simulink model "main"  (R2024a)
settings: Solver=VariableStepAuto  StartTime=0.0  StopTime=1  MaxStep=1e-4  RelTol=1e-3
InitFcn:
  | parametros
values from neighbouring files (symbols this model uses):
  alpha_cu = 3.9 *10^-3    (= 0.0039)    [parametros.m]
  b_l = 0.1    [parametros.m]
  b_m = 1.5 * 10^-5    (= 1.5e-05)    [parametros.m]
  C_ts = 0.818    [parametros.m]
  J_l = (m*l_cm^2 + J_cm) + (m_l * l_l^2)    (= 0.0833)    [parametros.m]
  J_m = 1.4 * 10^-5    (= 1.4e-05)    [parametros.m]
  k_l = m * g * l_cm + m_l * g * l_l    (= 2.4516625)    [parametros.m]
  L_d = 6.6 * 10^-3    (= 0.0066)    [parametros.m]
  L_ls = 0.8 * 10^-3    (= 0.0008)    [parametros.m]
  L_q = 5.8 * 10^-3    (= 0.0058)    [parametros.m]
  lambda_m = 0.016    [parametros.m]
  P_p = 3    [parametros.m]
  r = 120    [parametros.m]
  R_s_40 = 1.02    [parametros.m]
  R_ts_amb = 146.7    [parametros.m]
  Temp_s_ref = 40    [parametros.m]
(part 2 of 3)

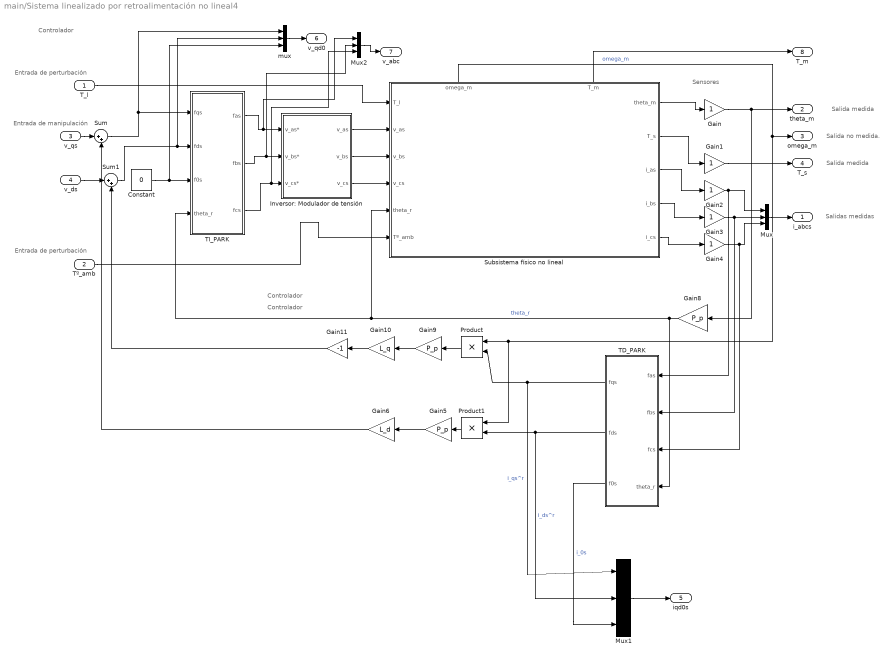
== system main/Sistema linealizado por retroalimentación no lineal4 ==
  note: Entrada de perturbación
  note: Entrada de manipulación
  note: Entrada de perturbación
  note: Controlador
  note: Salida medida
  note: Controlador
  note: Sensores
  note: Salida medida
  note: Salidas medidas
  note: Salida no medida.
  note: Controlador
  T_l : Inport
  Tº_amb : Inport  Port=2
  v_qs : Inport  Port=3
  v_ds : Inport  Port=4
  Constant : Constant  Value=0
  Gain{,1..4} (5 alike) : Gain
  Gain10 : Gain  Gain=L_q
  Gain11 : Gain  Gain=-1
  Gain5 : Gain  Gain=P_p
  Gain6 : Gain  Gain=L_d
  Gain8 : Gain  Gain=P_p
  Gain9 : Gain  Gain=P_p
  Inversor: Modulador de tensión : Subsystem
  Mux : Mux  Inputs=3
  Mux1 : Mux  Inputs=3
  Mux2 : Mux  Inputs=3
  Product : Product
  Product1 : Product
  "Subsistema físico no lineal " : Subsystem
      settings: PortSchema="{\"entries\":[{\"content\":{\"sides\":[{\"content\":{\"connectorIds\":[\"In1\",\"In2\",\"In3\",\"In4\",\"In5\",\"In6\"]},\"type\":\"ConnectorPlacement.EquallySpacedRectSide\",\"uuid\":\"df16c937-5b0d-437b-9581-4e7e4443d731\"},{\"content\":{\"connectorIds\":[\"Out1\",\"Out2\",\"Out3\",\"Out4\",\"Out5\"],\"side\":\"RIGHT\"},\"type\":\"ConnectorPlacement.EquallySpacedRectSide\",\"uuid\":\"58799b56-1bb2-4861-ad63-3fa3f8181ad5\"},{\"content\":{\"connectorIds\":[\"Out6\",\"Out7\"],\"side\":\"TOP\"},\"type\":\"ConnectorPlacement.EquallySpacedRectSide\",\"uuid\":\"9d658df7-49d2-4fa1-a84c-b158d9dac98e\"}]},\"type\":\"ConnectorPlacement.EquallySpacedConnector\",\"uuid\":\"4e139d46-6a94-417e-9cad-9c9676c83a39\"}],\"packageUris\":[\"http://schema.mathworks.com/mf0/Connector/R2020b\"],\"version\":\"1.0\"}"
  Sum : Sum  Inputs=|++
  Sum1 : Sum  Inputs=|++
  TD_PARK : MATLAB Function  TreatAsAtomicUnit=on
  TI_PARK : MATLAB Function  TreatAsAtomicUnit=on
  mux : Mux  Inputs=3
  i_abcs : Outport
  theta_m : Outport  Port=2
  omega_m : Outport  Port=3
  T_s : Outport  Port=4
  iqd0s : Outport  Port=5
  v_qd0 : Outport  Port=6
  v_abc : Outport  Port=7
  T_m : Outport  Port=8
  wires:
  T_l/1 -> "Subsistema físico no lineal "/1(T_l)
  "Subsistema físico no lineal "/2(T_s) -> Gain1/1
  "Subsistema físico no lineal "/1(theta_m) -> Gain/1
  Tº_amb/1 -> "Subsistema físico no lineal "/6(Tº_amb)
  "Subsistema físico no lineal "/4(i_bs) -> Gain3/1
  "Subsistema físico no lineal "/5(i_cs) -> Gain4/1
  "Subsistema físico no lineal "/3(i_as) -> Gain2/1
  Gain2/1 -> TD_PARK/1(fas), Mux/1
  Gain3/1 -> TD_PARK/2(fbs), Mux/2
  Gain4/1 -> TD_PARK/3(fcs), Mux/3
  Mux/1 -> i_abcs/1
  Gain/1 -> Gain8/1, theta_m/1
  "Subsistema físico no lineal "/6(omega_m) -> omega_m/1, Product1/1, Product/1  "omega_m"
  Gain1/1 -> T_s/1
  Gain8/1 -> "Subsistema físico no lineal "/5(theta_r), TI_PARK/4(theta_r), TD_PARK/4(theta_r)  "theta_r"
  TD_PARK/1(fqs) -> Mux1/1, Product/2  "i_qs^r"
  Product/1 -> Gain9/1
  Gain9/1 -> Gain10/1
  Gain10/1 -> Gain11/1
  Constant/1 -> TI_PARK/3(f0s), mux/3
  Inversor: Modulador de tensión/1(v_as) -> "Subsistema físico no lineal "/2(v_as)
  Inversor: Modulador de tensión/2(v_bs) -> "Subsistema físico no lineal "/3(v_bs)
  Inversor: Modulador de tensión/3(v_cs) -> "Subsistema físico no lineal "/4(v_cs)
  TI_PARK/1(fas) -> Mux2/1, Inversor: Modulador de tensión/1(v_as*)
  TI_PARK/2(fbs) -> Mux2/2, Inversor: Modulador de tensión/2(v_bs*)
  TI_PARK/3(fcs) -> Mux2/3, Inversor: Modulador de tensión/3(v_cs*)
  TD_PARK/2(fds) -> Mux1/2, Product1/2  "i_ds^r"
  TD_PARK/3(f0s) -> Mux1/3  "i_0s"
  Product1/1 -> Gain5/1
  Gain5/1 -> Gain6/1
  Mux1/1 -> iqd0s/1
  mux/1 -> v_qd0/1
  Mux2/1 -> v_abc/1
  "Subsistema físico no lineal "/7(T_m) -> T_m/1
  Gain11/1 -> Sum1/2
  v_qs/1 -> Sum/1
  Sum/1 -> TI_PARK/1(fqs), mux/1
  Gain6/1 -> Sum/2
  v_ds/1 -> Sum1/1
  Sum1/1 -> mux/2, TI_PARK/2(fds)

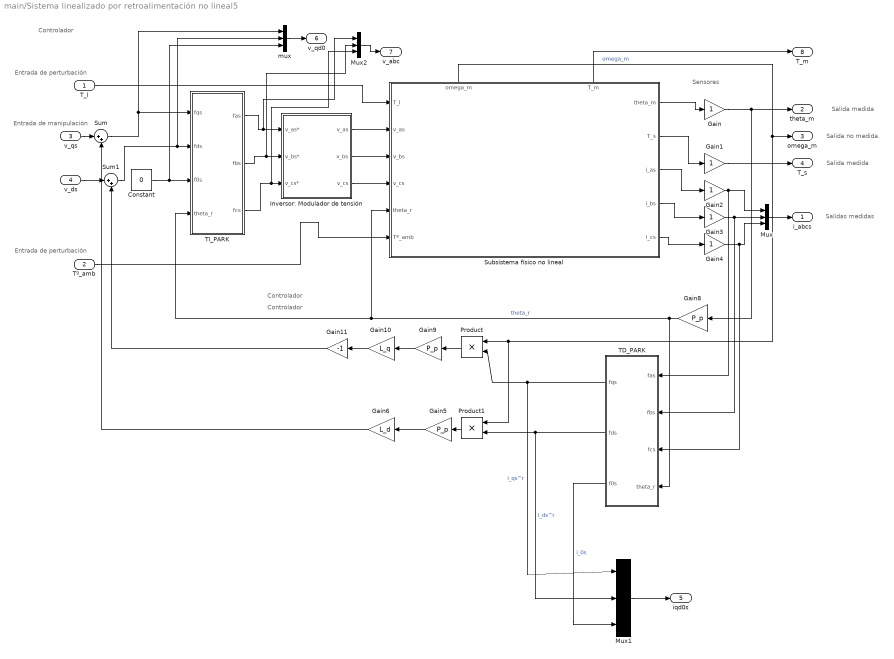
== system main/Sistema linealizado por retroalimentación no lineal5 ==
  note: Entrada de perturbación
  note: Entrada de manipulación
  note: Entrada de perturbación
  note: Controlador
  note: Salida medida
  note: Controlador
  note: Sensores
  note: Salida medida
  note: Salidas medidas
  note: Salida no medida.
  note: Controlador
  T_l : Inport
  Tº_amb : Inport  Port=2
  v_qs : Inport  Port=3
  v_ds : Inport  Port=4
  Constant : Constant  Value=0
  Gain{,1..4} (5 alike) : Gain
  Gain10 : Gain  Gain=L_q
  Gain11 : Gain  Gain=-1
  Gain5 : Gain  Gain=P_p
  Gain6 : Gain  Gain=L_d
  Gain8 : Gain  Gain=P_p
  Gain9 : Gain  Gain=P_p
  Inversor: Modulador de tensión : Subsystem
  Mux : Mux  Inputs=3
  Mux1 : Mux  Inputs=3
  Mux2 : Mux  Inputs=3
  Product : Product
  Product1 : Product
  "Subsistema físico no lineal " : Subsystem
      settings: PortSchema="{\"entries\":[{\"content\":{\"sides\":[{\"content\":{\"connectorIds\":[\"In1\",\"In2\",\"In3\",\"In4\",\"In5\",\"In6\"]},\"type\":\"ConnectorPlacement.EquallySpacedRectSide\",\"uuid\":\"df16c937-5b0d-437b-9581-4e7e4443d731\"},{\"content\":{\"connectorIds\":[\"Out1\",\"Out2\",\"Out3\",\"Out4\",\"Out5\"],\"side\":\"RIGHT\"},\"type\":\"ConnectorPlacement.EquallySpacedRectSide\",\"uuid\":\"58799b56-1bb2-4861-ad63-3fa3f8181ad5\"},{\"content\":{\"connectorIds\":[\"Out6\",\"Out7\"],\"side\":\"TOP\"},\"type\":\"ConnectorPlacement.EquallySpacedRectSide\",\"uuid\":\"9d658df7-49d2-4fa1-a84c-b158d9dac98e\"}]},\"type\":\"ConnectorPlacement.EquallySpacedConnector\",\"uuid\":\"4e139d46-6a94-417e-9cad-9c9676c83a39\"}],\"packageUris\":[\"http://schema.mathworks.com/mf0/Connector/R2020b\"],\"version\":\"1.0\"}"
  Sum : Sum  Inputs=|++
  Sum1 : Sum  Inputs=|++
  TD_PARK : MATLAB Function  TreatAsAtomicUnit=on
  TI_PARK : MATLAB Function  TreatAsAtomicUnit=on
  mux : Mux  Inputs=3
  i_abcs : Outport
  theta_m : Outport  Port=2
  omega_m : Outport  Port=3
  T_s : Outport  Port=4
  iqd0s : Outport  Port=5
  v_qd0 : Outport  Port=6
  v_abc : Outport  Port=7
  T_m : Outport  Port=8
  wires:
  T_l/1 -> "Subsistema físico no lineal "/1(T_l)
  "Subsistema físico no lineal "/2(T_s) -> Gain1/1
  "Subsistema físico no lineal "/1(theta_m) -> Gain/1
  Tº_amb/1 -> "Subsistema físico no lineal "/6(Tº_amb)
  "Subsistema físico no lineal "/4(i_bs) -> Gain3/1
  "Subsistema físico no lineal "/5(i_cs) -> Gain4/1
  "Subsistema físico no lineal "/3(i_as) -> Gain2/1
  Gain2/1 -> TD_PARK/1(fas), Mux/1
  Gain3/1 -> TD_PARK/2(fbs), Mux/2
  Gain4/1 -> TD_PARK/3(fcs), Mux/3
  Mux/1 -> i_abcs/1
  Gain/1 -> Gain8/1, theta_m/1
  "Subsistema físico no lineal "/6(omega_m) -> omega_m/1, Product1/1, Product/1  "omega_m"
  Gain1/1 -> T_s/1
  Gain8/1 -> "Subsistema físico no lineal "/5(theta_r), TI_PARK/4(theta_r), TD_PARK/4(theta_r)  "theta_r"
  TD_PARK/1(fqs) -> Mux1/1, Product/2  "i_qs^r"
  Product/1 -> Gain9/1
  Gain9/1 -> Gain10/1
  Gain10/1 -> Gain11/1
  Constant/1 -> TI_PARK/3(f0s), mux/3
  Inversor: Modulador de tensión/1(v_as) -> "Subsistema físico no lineal "/2(v_as)
  Inversor: Modulador de tensión/2(v_bs) -> "Subsistema físico no lineal "/3(v_bs)
  Inversor: Modulador de tensión/3(v_cs) -> "Subsistema físico no lineal "/4(v_cs)
  TI_PARK/1(fas) -> Mux2/1, Inversor: Modulador de tensión/1(v_as*)
  TI_PARK/2(fbs) -> Mux2/2, Inversor: Modulador de tensión/2(v_bs*)
  TI_PARK/3(fcs) -> Mux2/3, Inversor: Modulador de tensión/3(v_cs*)
  TD_PARK/2(fds) -> Mux1/2, Product1/2  "i_ds^r"
  TD_PARK/3(f0s) -> Mux1/3  "i_0s"
  Product1/1 -> Gain5/1
  Gain5/1 -> Gain6/1
  Mux1/1 -> iqd0s/1
  mux/1 -> v_qd0/1
  Mux2/1 -> v_abc/1
  "Subsistema físico no lineal "/7(T_m) -> T_m/1
  Gain11/1 -> Sum1/2
  v_qs/1 -> Sum/1
  Sum/1 -> TI_PARK/1(fqs), mux/1
  Gain6/1 -> Sum/2
  v_ds/1 -> Sum1/1
  Sum1/1 -> mux/2, TI_PARK/2(fds)

== system main/Sistema completo/Subsistema físico no lineal ==
  T_l : Inport
  v_qs^r : Inport  Port=2
  v_ds^r : Inport  Port=3
  v_0s^r : Inport  Port=4
  Tº_amb : Inport  Port=5
  Subsistema electromagnético : Subsystem
  Subsistema mecánico completo : Subsystem
  Subsistema térmico : Subsystem
  theta_m : Outport
  omega_m : Outport  Port=2
  T_s : Outport  Port=3
  i_qs^r : Outport  Port=4
  i_ds^r : Outport  Port=5
  i_0s^r : Outport  Port=6
  wires:
  Subsistema electromagnético/4(T_m) -> Subsistema mecánico completo/1(T_m)
  v_ds^r/1 -> Subsistema electromagnético/2(v_ds^r)
  Subsistema electromagnético/1(i_0s^r) -> Subsistema térmico/3(i_0s^r), i_0s^r/1
  Subsistema mecánico completo/2(omega_m(t)) -> omega_m/1, Subsistema electromagnético/4(omega_m)
  Subsistema electromagnético/3(i_qs^r) -> Subsistema térmico/1(i_qs^r), i_qs^r/1
  Subsistema electromagnético/2(i_ds^r) -> Subsistema térmico/2(i_ds^r), i_ds^r/1
  Subsistema térmico/2(r_s) -> Subsistema electromagnético/5(r_s)
  Subsistema térmico/1(T_s) -> T_s/1
  T_l/1 -> Subsistema mecánico completo/2(T_l)
  v_qs^r/1 -> Subsistema electromagnético/1(v_qs^r)
  v_0s^r/1 -> Subsistema electromagnético/3(v_0s^r)
  Subsistema mecánico completo/1(theta_m(t)) -> theta_m/1
  Tº_amb/1 -> Subsistema térmico/4(Tº_amb)

== system main/Sistema linealizado por retroalimentación no lineal/Inversor: Modulador de tensión ==
  v_as* : Inport
  v_bs* : Inport  Port=2
  v_cs* : Inport  Port=3
  Gain5 : Gain
  Gain6 : Gain
  Gain7 : Gain
  v_as : Outport
  v_bs : Outport  Port=2
  v_cs : Outport  Port=3
  wires:
  v_as*/1 -> Gain5/1
  Gain5/1 -> v_as/1
  v_cs*/1 -> Gain7/1
  v_bs*/1 -> Gain6/1
  Gain7/1 -> v_cs/1
  Gain6/1 -> v_bs/1

== system main/Sistema linealizado por retroalimentación no lineal/Subsistema físico no lineal  ==
  T_l : Inport
  v_as : Inport  Port=2
  v_bs : Inport  Port=3
  v_cs : Inport  Port=4
  theta_r : Inport  Port=5
  Tº_amb : Inport  Port=6
  Subsistema electromagnético : Subsystem
  Subsistema mecánico completo : Subsystem
  Subsistema térmico : Subsystem
  TD_PARK : MATLAB Function  TreatAsAtomicUnit=on
  TI_PARK : MATLAB Function  TreatAsAtomicUnit=on
  theta_m : Outport
  T_s : Outport  Port=2
  i_as : Outport  Port=3
  i_bs : Outport  Port=4
  i_cs : Outport  Port=5
  omega_m : Outport  Port=6
  wires:
  theta_r/1 -> TI_PARK/4(theta_r), TD_PARK/4(theta_r)
  TI_PARK/2(fbs) -> i_bs/1
  v_cs/1 -> TD_PARK/3(fcs)
  v_as/1 -> TD_PARK/1(fas)
  TI_PARK/3(fcs) -> i_cs/1
  v_bs/1 -> TD_PARK/2(fbs)
  TI_PARK/1(fas) -> i_as/1
  TD_PARK/1(fqs) -> Subsistema electromagnético/1(v_qs^r)
  TD_PARK/2(fds) -> Subsistema electromagnético/2(v_ds^r)
  TD_PARK/3(f0s) -> Subsistema electromagnético/3(v_0s^r)
  Subsistema mecánico completo/2(omega_m(t)) -> Subsistema electromagnético/4(omega_m), omega_m/1
  Subsistema térmico/2(r_s) -> Subsistema electromagnético/5(r_s)
  Subsistema electromagnético/2(i_ds^r) -> Subsistema térmico/2(i_ds^r), TI_PARK/2(fds)
  Subsistema electromagnético/3(i_qs^r) -> Subsistema térmico/1(i_qs^r), TI_PARK/1(fqs)
  Subsistema electromagnético/1(i_0s^r) -> Subsistema térmico/3(i_0s^r), TI_PARK/3(f0s)
  Subsistema electromagnético/4(T_m) -> Subsistema mecánico completo/1(T_m)
  T_l/1 -> Subsistema mecánico completo/2(T_l)
  Tº_amb/1 -> Subsistema térmico/4(Tº_amb)
  Subsistema térmico/1(T_s) -> T_s/1
  Subsistema mecánico completo/1(theta_m(t)) -> theta_m/1

== system main/Sistema linealizado por retroalimentación no lineal1/Inversor: Modulador de tensión ==
  v_as* : Inport
  v_bs* : Inport  Port=2
  v_cs* : Inport  Port=3
  Gain5 : Gain
  Gain6 : Gain
  Gain7 : Gain
  v_as : Outport
  v_bs : Outport  Port=2
  v_cs : Outport  Port=3
  wires:
  v_as*/1 -> Gain5/1
  Gain5/1 -> v_as/1
  v_cs*/1 -> Gain7/1
  v_bs*/1 -> Gain6/1
  Gain7/1 -> v_cs/1
  Gain6/1 -> v_bs/1

== system main/Sistema linealizado por retroalimentación no lineal1/Subsistema físico no lineal  ==
  T_l : Inport
  v_as : Inport  Port=2
  v_bs : Inport  Port=3
  v_cs : Inport  Port=4
  theta_r : Inport  Port=5
  Tº_amb : Inport  Port=6
  Subsistema electromagnético : Subsystem
  Subsistema mecánico completo : Subsystem
  Subsistema térmico : Subsystem
  TD_PARK : MATLAB Function  TreatAsAtomicUnit=on
  TI_PARK : MATLAB Function  TreatAsAtomicUnit=on
  theta_m : Outport
  T_s : Outport  Port=2
  i_as : Outport  Port=3
  i_bs : Outport  Port=4
  i_cs : Outport  Port=5
  omega_m : Outport  Port=6
  T_m : Outport  Port=7
  wires:
  theta_r/1 -> TI_PARK/4(theta_r), TD_PARK/4(theta_r)
  TI_PARK/2(fbs) -> i_bs/1
  v_cs/1 -> TD_PARK/3(fcs)
  v_as/1 -> TD_PARK/1(fas)
  TI_PARK/3(fcs) -> i_cs/1
  v_bs/1 -> TD_PARK/2(fbs)
  TI_PARK/1(fas) -> i_as/1
  TD_PARK/1(fqs) -> Subsistema electromagnético/1(v_qs^r)
  TD_PARK/2(fds) -> Subsistema electromagnético/2(v_ds^r)
  TD_PARK/3(f0s) -> Subsistema electromagnético/3(v_0s^r)
  Subsistema mecánico completo/2(omega_m(t)) -> Subsistema electromagnético/4(omega_m), omega_m/1
  Subsistema térmico/2(r_s) -> Subsistema electromagnético/5(r_s)
  Subsistema electromagnético/2(i_ds^r) -> Subsistema térmico/2(i_ds^r), TI_PARK/2(fds)
  Subsistema electromagnético/3(i_qs^r) -> Subsistema térmico/1(i_qs^r), TI_PARK/1(fqs)
  Subsistema electromagnético/1(i_0s^r) -> Subsistema térmico/3(i_0s^r), TI_PARK/3(f0s)
  Subsistema electromagnético/4(T_m) -> Subsistema mecánico completo/1(T_m), T_m/1
  T_l/1 -> Subsistema mecánico completo/2(T_l)
  Tº_amb/1 -> Subsistema térmico/4(Tº_amb)
  Subsistema térmico/1(T_s) -> T_s/1
  Subsistema mecánico completo/1(theta_m(t)) -> theta_m/1

== system main/Sistema linealizado por retroalimentación no lineal2/Inversor: Modulador de tensión ==
  v_as* : Inport
  v_bs* : Inport  Port=2
  v_cs* : Inport  Port=3
  Gain5 : Gain
  Gain6 : Gain
  Gain7 : Gain
  v_as : Outport
  v_bs : Outport  Port=2
  v_cs : Outport  Port=3
  wires:
  v_as*/1 -> Gain5/1
  Gain5/1 -> v_as/1
  v_cs*/1 -> Gain7/1
  v_bs*/1 -> Gain6/1
  Gain7/1 -> v_cs/1
  Gain6/1 -> v_bs/1

== system main/Sistema linealizado por retroalimentación no lineal2/Subsistema físico no lineal  ==
  T_l : Inport
  v_as : Inport  Port=2
  v_bs : Inport  Port=3
  v_cs : Inport  Port=4
  theta_r : Inport  Port=5
  Tº_amb : Inport  Port=6
  Subsistema electromagnético : Subsystem
  Subsistema mecánico completo : Subsystem
  Subsistema térmico : Subsystem
  TD_PARK : MATLAB Function  TreatAsAtomicUnit=on
  TI_PARK : MATLAB Function  TreatAsAtomicUnit=on
  theta_m : Outport
  T_s : Outport  Port=2
  i_as : Outport  Port=3
  i_bs : Outport  Port=4
  i_cs : Outport  Port=5
  omega_m : Outport  Port=6
  T_m : Outport  Port=7
  wires:
  theta_r/1 -> TI_PARK/4(theta_r), TD_PARK/4(theta_r)
  TI_PARK/2(fbs) -> i_bs/1
  v_cs/1 -> TD_PARK/3(fcs)
  v_as/1 -> TD_PARK/1(fas)
  TI_PARK/3(fcs) -> i_cs/1
  v_bs/1 -> TD_PARK/2(fbs)
  TI_PARK/1(fas) -> i_as/1
  TD_PARK/1(fqs) -> Subsistema electromagnético/1(v_qs^r)
  TD_PARK/2(fds) -> Subsistema electromagnético/2(v_ds^r)
  TD_PARK/3(f0s) -> Subsistema electromagnético/3(v_0s^r)
  Subsistema mecánico completo/2(omega_m(t)) -> Subsistema electromagnético/4(omega_m), omega_m/1
  Subsistema térmico/2(r_s) -> Subsistema electromagnético/5(r_s)
  Subsistema electromagnético/2(i_ds^r) -> Subsistema térmico/2(i_ds^r), TI_PARK/2(fds)
  Subsistema electromagnético/3(i_qs^r) -> Subsistema térmico/1(i_qs^r), TI_PARK/1(fqs)
  Subsistema electromagnético/1(i_0s^r) -> Subsistema térmico/3(i_0s^r), TI_PARK/3(f0s)
  Subsistema electromagnético/4(T_m) -> Subsistema mecánico completo/1(T_m), T_m/1
  T_l/1 -> Subsistema mecánico completo/2(T_l)
  Tº_amb/1 -> Subsistema térmico/4(Tº_amb)
  Subsistema térmico/1(T_s) -> T_s/1
  Subsistema mecánico completo/1(theta_m(t)) -> theta_m/1

== system main/Sistema linealizado por retroalimentación no lineal3/Inversor: Modulador de tensión ==
  v_as* : Inport
  v_bs* : Inport  Port=2
  v_cs* : Inport  Port=3
  Gain5 : Gain
  Gain6 : Gain
  Gain7 : Gain
  v_as : Outport
  v_bs : Outport  Port=2
  v_cs : Outport  Port=3
  wires:
  v_as*/1 -> Gain5/1
  Gain5/1 -> v_as/1
  v_cs*/1 -> Gain7/1
  v_bs*/1 -> Gain6/1
  Gain7/1 -> v_cs/1
  Gain6/1 -> v_bs/1

== system main/Sistema linealizado por retroalimentación no lineal3/Subsistema físico no lineal  ==
  T_l : Inport
  v_as : Inport  Port=2
  v_bs : Inport  Port=3
  v_cs : Inport  Port=4
  theta_r : Inport  Port=5
  Tº_amb : Inport  Port=6
  Subsistema electromagnético : Subsystem
  Subsistema mecánico completo : Subsystem
  Subsistema térmico : Subsystem
  TD_PARK : MATLAB Function  TreatAsAtomicUnit=on
  TI_PARK : MATLAB Function  TreatAsAtomicUnit=on
  theta_m : Outport
  T_s : Outport  Port=2
  i_as : Outport  Port=3
  i_bs : Outport  Port=4
  i_cs : Outport  Port=5
  omega_m : Outport  Port=6
  T_m : Outport  Port=7
  wires:
  theta_r/1 -> TI_PARK/4(theta_r), TD_PARK/4(theta_r)
  TI_PARK/2(fbs) -> i_bs/1
  v_cs/1 -> TD_PARK/3(fcs)
  v_as/1 -> TD_PARK/1(fas)
  TI_PARK/3(fcs) -> i_cs/1
  v_bs/1 -> TD_PARK/2(fbs)
  TI_PARK/1(fas) -> i_as/1
  TD_PARK/1(fqs) -> Subsistema electromagnético/1(v_qs^r)
  TD_PARK/2(fds) -> Subsistema electromagnético/2(v_ds^r)
  TD_PARK/3(f0s) -> Subsistema electromagnético/3(v_0s^r)
  Subsistema mecánico completo/2(omega_m(t)) -> Subsistema electromagnético/4(omega_m), omega_m/1
  Subsistema térmico/2(r_s) -> Subsistema electromagnético/5(r_s)
  Subsistema electromagnético/2(i_ds^r) -> Subsistema térmico/2(i_ds^r), TI_PARK/2(fds)
  Subsistema electromagnético/3(i_qs^r) -> Subsistema térmico/1(i_qs^r), TI_PARK/1(fqs)
  Subsistema electromagnético/1(i_0s^r) -> Subsistema térmico/3(i_0s^r), TI_PARK/3(f0s)
  Subsistema electromagnético/4(T_m) -> Subsistema mecánico completo/1(T_m), T_m/1
  T_l/1 -> Subsistema mecánico completo/2(T_l)
  Tº_amb/1 -> Subsistema térmico/4(Tº_amb)
  Subsistema térmico/1(T_s) -> T_s/1
  Subsistema mecánico completo/1(theta_m(t)) -> theta_m/1

== system main/Sistema linealizado por retroalimentación no lineal4/Inversor: Modulador de tensión ==
  v_as* : Inport
  v_bs* : Inport  Port=2
  v_cs* : Inport  Port=3
  Gain5 : Gain
  Gain6 : Gain
  Gain7 : Gain
  v_as : Outport
  v_bs : Outport  Port=2
  v_cs : Outport  Port=3
  wires:
  v_as*/1 -> Gain5/1
  Gain5/1 -> v_as/1
  v_cs*/1 -> Gain7/1
  v_bs*/1 -> Gain6/1
  Gain7/1 -> v_cs/1
  Gain6/1 -> v_bs/1

== system main/Sistema linealizado por retroalimentación no lineal4/Subsistema físico no lineal  ==
  T_l : Inport
  v_as : Inport  Port=2
  v_bs : Inport  Port=3
  v_cs : Inport  Port=4
  theta_r : Inport  Port=5
  Tº_amb : Inport  Port=6
  Subsistema electromagnético : Subsystem
  Subsistema mecánico completo : Subsystem
  Subsistema térmico : Subsystem
  TD_PARK : MATLAB Function  TreatAsAtomicUnit=on
  TI_PARK : MATLAB Function  TreatAsAtomicUnit=on
  theta_m : Outport
  T_s : Outport  Port=2
  i_as : Outport  Port=3
  i_bs : Outport  Port=4
  i_cs : Outport  Port=5
  omega_m : Outport  Port=6
  T_m : Outport  Port=7
  wires:
  theta_r/1 -> TI_PARK/4(theta_r), TD_PARK/4(theta_r)
  TI_PARK/2(fbs) -> i_bs/1
  v_cs/1 -> TD_PARK/3(fcs)
  v_as/1 -> TD_PARK/1(fas)
  TI_PARK/3(fcs) -> i_cs/1
  v_bs/1 -> TD_PARK/2(fbs)
  TI_PARK/1(fas) -> i_as/1
  TD_PARK/1(fqs) -> Subsistema electromagnético/1(v_qs^r)
  TD_PARK/2(fds) -> Subsistema electromagnético/2(v_ds^r)
  TD_PARK/3(f0s) -> Subsistema electromagnético/3(v_0s^r)
  Subsistema mecánico completo/2(omega_m(t)) -> Subsistema electromagnético/4(omega_m), omega_m/1
  Subsistema térmico/2(r_s) -> Subsistema electromagnético/5(r_s)
  Subsistema electromagnético/2(i_ds^r) -> Subsistema térmico/2(i_ds^r), TI_PARK/2(fds)
  Subsistema electromagnético/3(i_qs^r) -> Subsistema térmico/1(i_qs^r), TI_PARK/1(fqs)
  Subsistema electromagnético/1(i_0s^r) -> Subsistema térmico/3(i_0s^r), TI_PARK/3(f0s)
  Subsistema electromagnético/4(T_m) -> Subsistema mecánico completo/1(T_m), T_m/1
  T_l/1 -> Subsistema mecánico completo/2(T_l)
  Tº_amb/1 -> Subsistema térmico/4(Tº_amb)
  Subsistema térmico/1(T_s) -> T_s/1
  Subsistema mecánico completo/1(theta_m(t)) -> theta_m/1

== system main/Sistema linealizado por retroalimentación no lineal5/Inversor: Modulador de tensión ==
  v_as* : Inport
  v_bs* : Inport  Port=2
  v_cs* : Inport  Port=3
  Gain5 : Gain
  Gain6 : Gain
  Gain7 : Gain
  v_as : Outport
  v_bs : Outport  Port=2
  v_cs : Outport  Port=3
  wires:
  v_as*/1 -> Gain5/1
  Gain5/1 -> v_as/1
  v_cs*/1 -> Gain7/1
  v_bs*/1 -> Gain6/1
  Gain7/1 -> v_cs/1
  Gain6/1 -> v_bs/1

== system main/Sistema linealizado por retroalimentación no lineal5/Subsistema físico no lineal  ==
  T_l : Inport
  v_as : Inport  Port=2
  v_bs : Inport  Port=3
  v_cs : Inport  Port=4
  theta_r : Inport  Port=5
  Tº_amb : Inport  Port=6
  Subsistema electromagnético : Subsystem
  Subsistema mecánico completo : Subsystem
  Subsistema térmico : Subsystem
  TD_PARK : MATLAB Function  TreatAsAtomicUnit=on
  TI_PARK : MATLAB Function  TreatAsAtomicUnit=on
  theta_m : Outport
  T_s : Outport  Port=2
  i_as : Outport  Port=3
  i_bs : Outport  Port=4
  i_cs : Outport  Port=5
  omega_m : Outport  Port=6
  T_m : Outport  Port=7
  wires:
  theta_r/1 -> TI_PARK/4(theta_r), TD_PARK/4(theta_r)
  TI_PARK/2(fbs) -> i_bs/1
  v_cs/1 -> TD_PARK/3(fcs)
  v_as/1 -> TD_PARK/1(fas)
  TI_PARK/3(fcs) -> i_cs/1
  v_bs/1 -> TD_PARK/2(fbs)
  TI_PARK/1(fas) -> i_as/1
  TD_PARK/1(fqs) -> Subsistema electromagnético/1(v_qs^r)
  TD_PARK/2(fds) -> Subsistema electromagnético/2(v_ds^r)
  TD_PARK/3(f0s) -> Subsistema electromagnético/3(v_0s^r)
  Subsistema mecánico completo/2(omega_m(t)) -> Subsistema electromagnético/4(omega_m), omega_m/1
  Subsistema térmico/2(r_s) -> Subsistema electromagnético/5(r_s)
  Subsistema electromagnético/2(i_ds^r) -> Subsistema térmico/2(i_ds^r), TI_PARK/2(fds)
  Subsistema electromagnético/3(i_qs^r) -> Subsistema térmico/1(i_qs^r), TI_PARK/1(fqs)
  Subsistema electromagnético/1(i_0s^r) -> Subsistema térmico/3(i_0s^r), TI_PARK/3(f0s)
  Subsistema electromagnético/4(T_m) -> Subsistema mecánico completo/1(T_m), T_m/1
  T_l/1 -> Subsistema mecánico completo/2(T_l)
  Tº_amb/1 -> Subsistema térmico/4(Tº_amb)
  Subsistema térmico/1(T_s) -> T_s/1
  Subsistema mecánico completo/1(theta_m(t)) -> theta_m/1

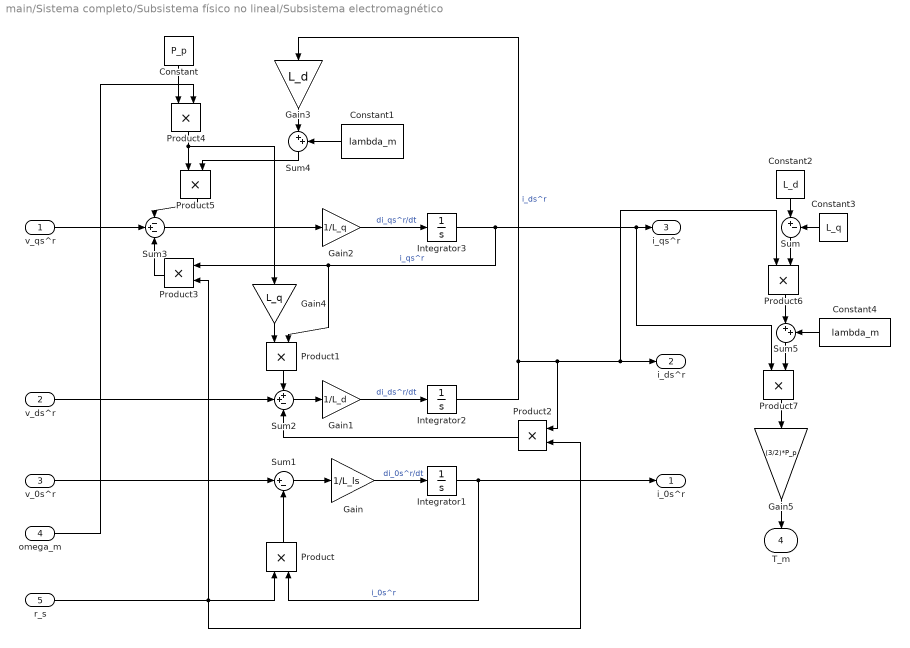
== system main/Sistema completo/Subsistema físico no lineal/Subsistema electromagnético ==
  v_qs^r : Inport
  v_ds^r : Inport  Port=2
  v_0s^r : Inport  Port=3
  omega_m : Inport  Port=4
  r_s : Inport  Port=5
  Constant : Constant  Value=P_p
  Constant1 : Constant  Value=lambda_m
  Constant2 : Constant  Value=L_d
  Constant3 : Constant  Value=L_q
  Constant4 : Constant  Value=lambda_m
  Gain : Gain  Gain=1/L_ls
  Gain1 : Gain  Gain=1/L_d
  Gain2 : Gain  Gain=1/L_q
  Gain3 : Gain  Gain=L_d
  Gain4 : Gain  Gain=L_q
  Gain5 : Gain  Gain=(3/2)*P_p
  Integrator1 : Integrator
  Integrator2 : Integrator
  Integrator3 : Integrator
  Product{,1..7} (8 alike) : Product
  Sum : Sum  Inputs=|+-
  Sum1 : Sum  Inputs=|+-
  Sum2 : Sum  Inputs=++-
  Sum3 : Sum  Inputs=-+-
  Sum4 : Sum  Inputs=|++
  Sum5 : Sum  Inputs=|++
  i_0s^r : Outport
  i_ds^r : Outport  Port=2
  i_qs^r : Outport  Port=3
  T_m : Outport  Port=4
  wires:
  Integrator1/1 -> i_0s^r/1, Product/2  "i_0s^r"
  r_s/1 -> Product3/2, Product2/2, Product/1
  Sum1/1 -> Gain/1
  Product/1 -> Sum1/2
  Gain/1 -> Integrator1/1  "di_0s^r/dt"
  v_0s^r/1 -> Sum1/1
  Integrator2/1 -> Gain3/1, Product2/1, Product6/1, i_ds^r/1  "i_ds^r"
  Gain1/1 -> Integrator2/1  "di_ds^r/dt"
  Sum2/1 -> Gain1/1
  Integrator3/1 -> Product1/2, Product3/1, Product7/1, i_qs^r/1  "i_qs^r"
  Gain2/1 -> Integrator3/1  "di_qs^r/dt"
  Product3/1 -> Sum3/3
  v_qs^r/1 -> Sum3/2
  Constant/1 -> Product4/1
  omega_m/1 -> Product4/2
  Product4/1 -> Gain4/1, Product5/1
  Gain3/1 -> Sum4/1
  Sum4/1 -> Product5/2
  Constant1/1 -> Sum4/2
  Product5/1 -> Sum3/1
  Sum3/1 -> Gain2/1
  v_ds^r/1 -> Sum2/2
  Gain4/1 -> Product1/1
  Product1/1 -> Sum2/1
  Product2/1 -> Sum2/3
  Constant2/1 -> Sum/1
  Constant3/1 -> Sum/2
  Sum/1 -> Product6/2
  Product6/1 -> Sum5/1
  Constant4/1 -> Sum5/2
  Sum5/1 -> Product7/2
  Product7/1 -> Gain5/1
  Gain5/1 -> T_m/1

== system main/Sistema completo/Subsistema físico no lineal/Subsistema mecánico completo ==
  T_m : Inport
  T_l : Inport  Port=2
  Gain : Gain  Gain=b_m + b_l / (r^2)
  Gain1 : Gain  Gain=1/r
  Gain2 : Gain  Gain=1/(J_m + J_l / r^2)
  Sum : Sum  Inputs=-+-
  omega_m(0) = 0 : Integrator
  theta_m(0) = 0 : Integrator
  theta_m(t) : Outport
  omega_m(t) : Outport  Port=2
  wires:
  Gain2/1 -> omega_m(0) = 0/1  "domega_m(t)/dt"
  Gain1/1 -> Sum/1
  theta_m(0) = 0/1 -> theta_m(t)/1  "theta_m(t)"
  omega_m(0) = 0/1 -> omega_m(t)/1, Gain/1, theta_m(0) = 0/1  "omega_m(t)"
  Sum/1 -> Gain2/1
  Gain/1 -> Sum/3
  T_l/1 -> Gain1/1
  T_m/1 -> Sum/2

== system main/Sistema completo/Subsistema físico no lineal/Subsistema térmico ==
  i_qs^r : Inport
  i_ds^r : Inport  Port=2
  i_0s^r : Inport  Port=3
  Tº_amb : Inport  Port=4
  Constant : Constant  Value=R_s_40
  Constant1 : Constant
  Constant2 : Constant  Value=Temp_s_ref
  Gain : Gain  Gain=2
  Gain1 : Gain  Gain=1.5
  Gain2 : Gain  Gain=1/C_ts
  Gain3 : Gain  Gain=1/(R_ts_amb)
  Gain4 : Gain  Gain=alpha_cu
  Integrator : Integrator
  Product : Product
  Product1 : Product
  Square : Math  Operator=square
  Square1 : Math  Operator=square
  Square2 : Math  Operator=square
  Sum : Sum  Inputs=+++
  Sum1 : Sum  Inputs=|+-
  Sum2 : Sum  Inputs=-+
  Sum3 : Sum  Inputs=|++
  Sum4 : Sum  Inputs=|+-
  T_s : Outport
  r_s : Outport  Port=2
  wires:
  Square1/1 -> Sum/2
  Square/1 -> Sum/1
  Gain/1 -> Sum/3
  Constant/1 -> Product1/2
  Sum/1 -> Product/1
  Gain1/1 -> Product/2
  Gain3/1 -> Sum1/2
  Sum1/1 -> Gain2/1
  Integrator/1 -> T_s/1, Sum4/1, Sum2/2  "T_s"
  Sum2/1 -> Gain3/1
  Constant1/1 -> Sum3/1
  Gain4/1 -> Sum3/2
  Sum3/1 -> Product1/1
  Square2/1 -> Gain/1
  Constant2/1 -> Sum4/2
  Sum4/1 -> Gain4/1
  Gain2/1 -> Integrator/1  "dT_s/dt"
  Product/1 -> Sum1/1
  i_qs^r/1 -> Square/1
  Tº_amb/1 -> Sum2/1
  i_0s^r/1 -> Square2/1
  i_ds^r/1 -> Square1/1
  Product1/1 -> Gain1/1, r_s/1

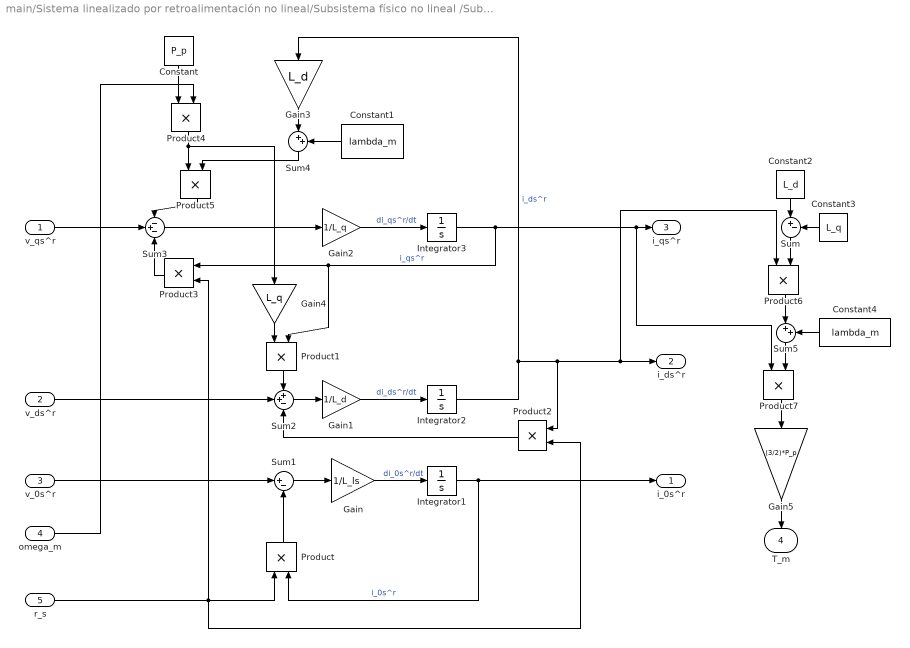
== system main/Sistema linealizado por retroalimentación no lineal/Subsistema físico no lineal /Subsistema electromagnético ==
  v_qs^r : Inport
  v_ds^r : Inport  Port=2
  v_0s^r : Inport  Port=3
  omega_m : Inport  Port=4
  r_s : Inport  Port=5
  Constant : Constant  Value=P_p
  Constant1 : Constant  Value=lambda_m
  Constant2 : Constant  Value=L_d
  Constant3 : Constant  Value=L_q
  Constant4 : Constant  Value=lambda_m
  Gain : Gain  Gain=1/L_ls
  Gain1 : Gain  Gain=1/L_d
  Gain2 : Gain  Gain=1/L_q
  Gain3 : Gain  Gain=L_d
  Gain4 : Gain  Gain=L_q
  Gain5 : Gain  Gain=(3/2)*P_p
  Integrator1 : Integrator
  Integrator2 : Integrator
  Integrator3 : Integrator
  Product{,1..7} (8 alike) : Product
  Sum : Sum  Inputs=|+-
  Sum1 : Sum  Inputs=|+-
  Sum2 : Sum  Inputs=++-
  Sum3 : Sum  Inputs=-+-
  Sum4 : Sum  Inputs=|++
  Sum5 : Sum  Inputs=|++
  i_0s^r : Outport
  i_ds^r : Outport  Port=2
  i_qs^r : Outport  Port=3
  T_m : Outport  Port=4
  wires:
  Integrator1/1 -> i_0s^r/1, Product/2  "i_0s^r"
  r_s/1 -> Product3/2, Product2/2, Product/1
  Sum1/1 -> Gain/1
  Product/1 -> Sum1/2
  Gain/1 -> Integrator1/1  "di_0s^r/dt"
  v_0s^r/1 -> Sum1/1
  Integrator2/1 -> Gain3/1, Product2/1, Product6/1, i_ds^r/1  "i_ds^r"
  Gain1/1 -> Integrator2/1  "di_ds^r/dt"
  Sum2/1 -> Gain1/1
  Integrator3/1 -> Product1/2, Product3/1, Product7/1, i_qs^r/1  "i_qs^r"
  Gain2/1 -> Integrator3/1  "di_qs^r/dt"
  Product3/1 -> Sum3/3
  v_qs^r/1 -> Sum3/2
  Constant/1 -> Product4/1
  omega_m/1 -> Product4/2
  Product4/1 -> Gain4/1, Product5/1
  Gain3/1 -> Sum4/1
  Sum4/1 -> Product5/2
  Constant1/1 -> Sum4/2
  Product5/1 -> Sum3/1
  Sum3/1 -> Gain2/1
  v_ds^r/1 -> Sum2/2
  Gain4/1 -> Product1/1
  Product1/1 -> Sum2/1
  Product2/1 -> Sum2/3
  Constant2/1 -> Sum/1
  Constant3/1 -> Sum/2
  Sum/1 -> Product6/2
  Product6/1 -> Sum5/1
  Constant4/1 -> Sum5/2
  Sum5/1 -> Product7/2
  Product7/1 -> Gain5/1
  Gain5/1 -> T_m/1

== system main/Sistema linealizado por retroalimentación no lineal/Subsistema físico no lineal /Subsistema mecánico completo ==
  T_m : Inport
  T_l : Inport  Port=2
  Gain : Gain  Gain=b_m + b_l / (r^2)
  Gain1 : Gain  Gain=1/r
  Gain2 : Gain  Gain=1/(J_m + J_l / r^2)
  Sum : Sum  Inputs=-+-
  omega_m(0) = 0 : Integrator
  theta_m(0) = 0 : Integrator
  theta_m(t) : Outport
  omega_m(t) : Outport  Port=2
  wires:
  Gain2/1 -> omega_m(0) = 0/1  "domega_m(t)/dt"
  Gain1/1 -> Sum/1
  theta_m(0) = 0/1 -> theta_m(t)/1  "theta_m(t)"
  omega_m(0) = 0/1 -> omega_m(t)/1, Gain/1, theta_m(0) = 0/1  "omega_m(t)"
  Sum/1 -> Gain2/1
  Gain/1 -> Sum/3
  T_l/1 -> Gain1/1
  T_m/1 -> Sum/2

== system main/Sistema linealizado por retroalimentación no lineal/Subsistema físico no lineal /Subsistema térmico ==
  i_qs^r : Inport
  i_ds^r : Inport  Port=2
  i_0s^r : Inport  Port=3
  Tº_amb : Inport  Port=4
  Constant : Constant  Value=R_s_40
  Constant1 : Constant
  Constant2 : Constant  Value=Temp_s_ref
  Gain : Gain  Gain=2
  Gain1 : Gain  Gain=1.5
  Gain2 : Gain  Gain=1/C_ts
  Gain3 : Gain  Gain=1/(R_ts_amb)
  Gain4 : Gain  Gain=alpha_cu
  Integrator : Integrator
  Product : Product
  Product1 : Product
  Square : Math  Operator=square
  Square1 : Math  Operator=square
  Square2 : Math  Operator=square
  Sum : Sum  Inputs=+++
  Sum1 : Sum  Inputs=|+-
  Sum2 : Sum  Inputs=-+
  Sum3 : Sum  Inputs=|++
  Sum4 : Sum  Inputs=|+-
  T_s : Outport
  r_s : Outport  Port=2
  wires:
  Square1/1 -> Sum/2
  Square/1 -> Sum/1
  Gain/1 -> Sum/3
  Constant/1 -> Product1/2
  Sum/1 -> Product/1
  Gain1/1 -> Product/2
  Gain3/1 -> Sum1/2
  Sum1/1 -> Gain2/1
  Integrator/1 -> T_s/1, Sum4/1, Sum2/2  "T_s"
  Sum2/1 -> Gain3/1
  Constant1/1 -> Sum3/1
  Gain4/1 -> Sum3/2
  Sum3/1 -> Product1/1
  Square2/1 -> Gain/1
  Constant2/1 -> Sum4/2
  Sum4/1 -> Gain4/1
  Gain2/1 -> Integrator/1  "dT_s/dt"
  Product/1 -> Sum1/1
  i_qs^r/1 -> Square/1
  Tº_amb/1 -> Sum2/1
  i_0s^r/1 -> Square2/1
  i_ds^r/1 -> Square1/1
  Product1/1 -> Gain1/1, r_s/1

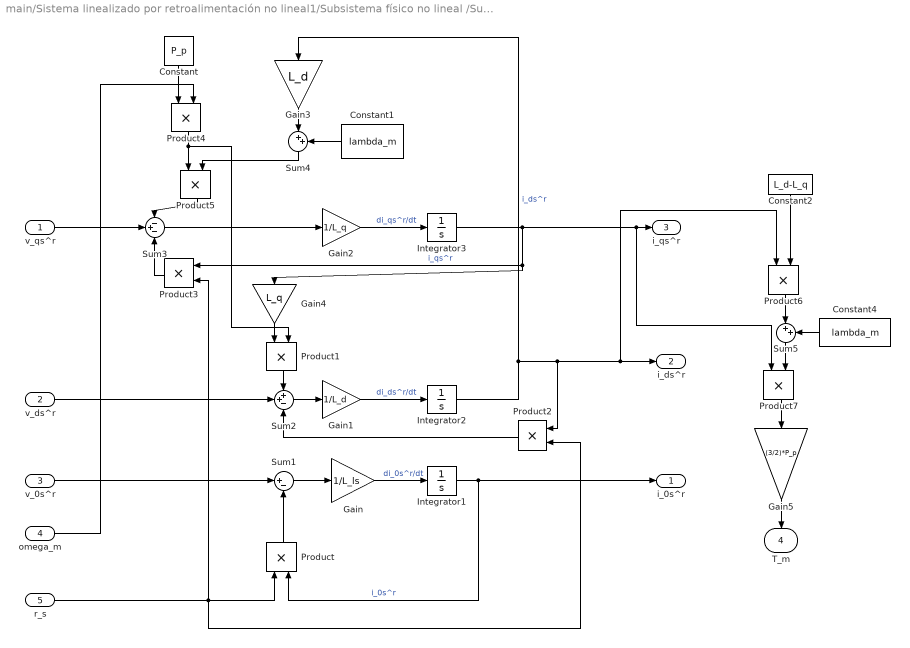
== system main/Sistema linealizado por retroalimentación no lineal1/Subsistema físico no lineal /Subsistema electromagnético ==
  v_qs^r : Inport
  v_ds^r : Inport  Port=2
  v_0s^r : Inport  Port=3
  omega_m : Inport  Port=4
  r_s : Inport  Port=5
  Constant : Constant  Value=P_p
  Constant1 : Constant  Value=lambda_m
  Constant2 : Constant  Value=L_d-L_q
  Constant4 : Constant  Value=lambda_m
  Gain : Gain  Gain=1/L_ls
  Gain1 : Gain  Gain=1/L_d
  Gain2 : Gain  Gain=1/L_q
  Gain3 : Gain  Gain=L_d
  Gain4 : Gain  Gain=L_q
  Gain5 : Gain  Gain=(3/2)*P_p
  Integrator1 : Integrator
  Integrator2 : Integrator
  Integrator3 : Integrator
  Product{,1..7} (8 alike) : Product
  Sum1 : Sum  Inputs=|+-
  Sum2 : Sum  Inputs=++-
  Sum3 : Sum  Inputs=-+-
  Sum4 : Sum  Inputs=|++
  Sum5 : Sum  Inputs=|++
  i_0s^r : Outport
  i_ds^r : Outport  Port=2
  i_qs^r : Outport  Port=3
  T_m : Outport  Port=4
  wires:
  Integrator1/1 -> i_0s^r/1, Product/2  "i_0s^r"
  r_s/1 -> Product3/2, Product2/2, Product/1
  Sum1/1 -> Gain/1
  Product/1 -> Sum1/2
  Gain/1 -> Integrator1/1  "di_0s^r/dt"
  v_0s^r/1 -> Sum1/1
  Integrator2/1 -> Gain3/1, Product2/1, Product6/1, i_ds^r/1  "i_ds^r"
  Gain1/1 -> Integrator2/1  "di_ds^r/dt"
  Sum2/1 -> Gain1/1
  Integrator3/1 -> Product3/1, Gain4/1, Product7/1, i_qs^r/1  "i_qs^r"
  Gain2/1 -> Integrator3/1  "di_qs^r/dt"
  Product3/1 -> Sum3/3
  v_qs^r/1 -> Sum3/2
  Constant/1 -> Product4/1
  omega_m/1 -> Product4/2
  Product4/1 -> Product1/2, Product5/1
  Gain3/1 -> Sum4/1
  Sum4/1 -> Product5/2
  Constant1/1 -> Sum4/2
  Product5/1 -> Sum3/1
  Sum3/1 -> Gain2/1
  v_ds^r/1 -> Sum2/2
  Gain4/1 -> Product1/1
  Product1/1 -> Sum2/1
  Product2/1 -> Sum2/3
  Product6/1 -> Sum5/1
  Constant4/1 -> Sum5/2
  Sum5/1 -> Product7/2
  Product7/1 -> Gain5/1
  Gain5/1 -> T_m/1
  Constant2/1 -> Product6/2

== system main/Sistema linealizado por retroalimentación no lineal1/Subsistema físico no lineal /Subsistema mecánico completo ==
  T_m : Inport
  T_l : Inport  Port=2
  Gain : Gain  Gain=b_m +( b_l / (r^2))
  Gain1 : Gain  Gain=1/r
  Gain2 : Gain  Gain=1/(J_m + J_l / (r^2))
  Sum : Sum  Inputs=-+-
  omega_m(0) = 0 : Integrator
  theta_m(0) = 0 : Integrator
  theta_m(t) : Outport
  omega_m(t) : Outport  Port=2
  wires:
  Gain2/1 -> omega_m(0) = 0/1  "domega_m(t)/dt"
  Gain1/1 -> Sum/1
  theta_m(0) = 0/1 -> theta_m(t)/1  "theta_m(t)"
  omega_m(0) = 0/1 -> omega_m(t)/1, Gain/1, theta_m(0) = 0/1  "omega_m(t)"
  Sum/1 -> Gain2/1
  Gain/1 -> Sum/3
  T_l/1 -> Gain1/1
  T_m/1 -> Sum/2

== system main/Sistema linealizado por retroalimentación no lineal1/Subsistema físico no lineal /Subsistema térmico ==
  i_qs^r : Inport
  i_ds^r : Inport  Port=2
  i_0s^r : Inport  Port=3
  Tº_amb : Inport  Port=4
  CI = 40ºC : Integrator  InitialCondition=40
  Constant : Constant
  Gain : Gain  Gain=1/C_ts
  Gain1 : Gain  Gain=2
  Gain2 : Gain  Gain=3/2
  Gain3 : Gain  Gain=1/R_ts_amb
  Gain4 : Gain  Gain=alpha_cu
  Gain5 : Gain  Gain=R_s_40
  Product : Product
  Square : Math  Operator=square
  Square1 : Math  Operator=square
  Square2 : Math  Operator=square
  Sum : Sum  Inputs=+++
  Sum1 : Sum  Inputs=|+-
  Sum2 : Sum  Inputs=|+-
  Sum3 : Sum  Inputs=|++
  T_s : Outport
  r_s : Outport  Port=2
  wires:
  CI = 40ºC/1 -> Sum2/2, T_s/1
  Gain/1 -> CI = 40ºC/1
  Sum1/1 -> Gain/1
  i_qs^r/1 -> Square/1
  i_ds^r/1 -> Square1/1
  i_0s^r/1 -> Square2/1
  Square2/1 -> Gain1/1
  Square/1 -> Sum/1
  Square1/1 -> Sum/2
  Gain1/1 -> Sum/3
  Gain5/1 -> r_s/1, Gain2/1
  Gain2/1 -> Product/2
  Sum/1 -> Product/1
  Product/1 -> Sum1/1
  Tº_amb/1 -> Sum2/1
  Sum2/1 -> Gain4/1, Gain3/1
  Gain3/1 -> Sum1/2
  Gain4/1 -> Sum3/1
  Constant/1 -> Sum3/2
  Sum3/1 -> Gain5/1

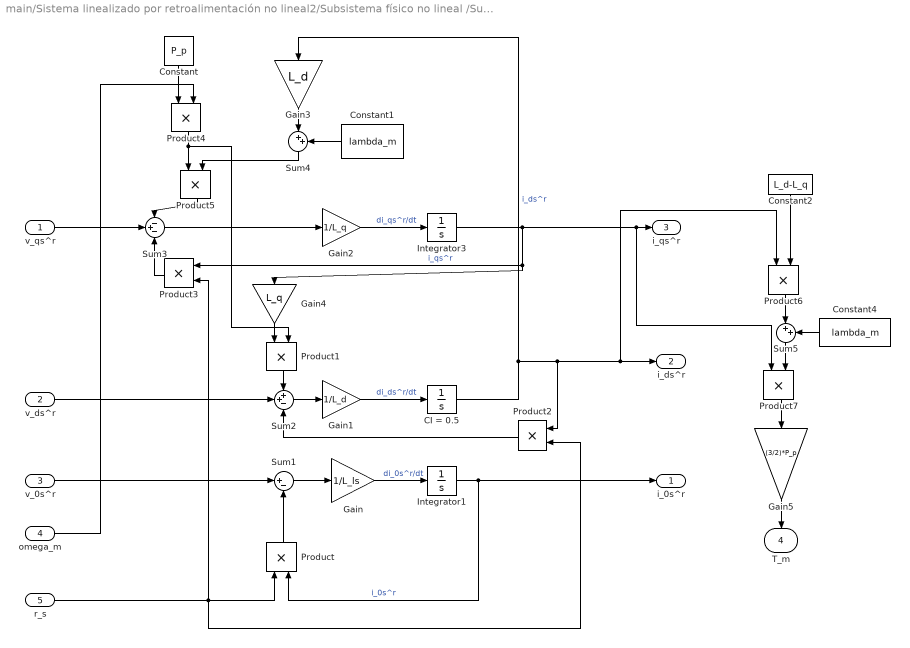
== system main/Sistema linealizado por retroalimentación no lineal2/Subsistema físico no lineal /Subsistema electromagnético ==
  v_qs^r : Inport
  v_ds^r : Inport  Port=2
  v_0s^r : Inport  Port=3
  omega_m : Inport  Port=4
  r_s : Inport  Port=5
  CI = 0.5 : Integrator  InitialCondition=0.5
  Constant : Constant  Value=P_p
  Constant1 : Constant  Value=lambda_m
  Constant2 : Constant  Value=L_d-L_q
  Constant4 : Constant  Value=lambda_m
  Gain : Gain  Gain=1/L_ls
  Gain1 : Gain  Gain=1/L_d
  Gain2 : Gain  Gain=1/L_q
  Gain3 : Gain  Gain=L_d
  Gain4 : Gain  Gain=L_q
  Gain5 : Gain  Gain=(3/2)*P_p
  Integrator1 : Integrator
  Integrator3 : Integrator
  Product{,1..7} (8 alike) : Product
  Sum1 : Sum  Inputs=|+-
  Sum2 : Sum  Inputs=++-
  Sum3 : Sum  Inputs=-+-
  Sum4 : Sum  Inputs=|++
  Sum5 : Sum  Inputs=|++
  i_0s^r : Outport
  i_ds^r : Outport  Port=2
  i_qs^r : Outport  Port=3
  T_m : Outport  Port=4
  wires:
  Integrator1/1 -> i_0s^r/1, Product/2  "i_0s^r"
  r_s/1 -> Product3/2, Product2/2, Product/1
  Sum1/1 -> Gain/1
  Product/1 -> Sum1/2
  Gain/1 -> Integrator1/1  "di_0s^r/dt"
  v_0s^r/1 -> Sum1/1
  CI = 0.5/1 -> Gain3/1, Product2/1, Product6/1, i_ds^r/1  "i_ds^r"
  Gain1/1 -> CI = 0.5/1  "di_ds^r/dt"
  Sum2/1 -> Gain1/1
  Integrator3/1 -> Product3/1, Gain4/1, Product7/1, i_qs^r/1  "i_qs^r"
  Gain2/1 -> Integrator3/1  "di_qs^r/dt"
  Product3/1 -> Sum3/3
  v_qs^r/1 -> Sum3/2
  Constant/1 -> Product4/1
  omega_m/1 -> Product4/2
  Product4/1 -> Product1/2, Product5/1
  Gain3/1 -> Sum4/1
  Sum4/1 -> Product5/2
  Constant1/1 -> Sum4/2
  Product5/1 -> Sum3/1
  Sum3/1 -> Gain2/1
  v_ds^r/1 -> Sum2/2
  Gain4/1 -> Product1/1
  Product1/1 -> Sum2/1
  Product2/1 -> Sum2/3
  Product6/1 -> Sum5/1
  Constant4/1 -> Sum5/2
  Sum5/1 -> Product7/2
  Product7/1 -> Gain5/1
  Gain5/1 -> T_m/1
  Constant2/1 -> Product6/2

== system main/Sistema linealizado por retroalimentación no lineal2/Subsistema físico no lineal /Subsistema mecánico completo ==
  T_m : Inport
  T_l : Inport  Port=2
  Gain : Gain  Gain=b_m +( b_l / (r^2))
  Gain1 : Gain  Gain=1/r
  Gain2 : Gain  Gain=1/(J_m + J_l / (r^2))
  Sum : Sum  Inputs=-+-
  omega_m(0) = 0 : Integrator
  theta_m(0) = 0 : Integrator
  theta_m(t) : Outport
  omega_m(t) : Outport  Port=2
  wires:
  Gain2/1 -> omega_m(0) = 0/1  "domega_m(t)/dt"
  Gain1/1 -> Sum/1
  theta_m(0) = 0/1 -> theta_m(t)/1  "theta_m(t)"
  omega_m(0) = 0/1 -> omega_m(t)/1, Gain/1, theta_m(0) = 0/1  "omega_m(t)"
  Sum/1 -> Gain2/1
  Gain/1 -> Sum/3
  T_l/1 -> Gain1/1
  T_m/1 -> Sum/2

== system main/Sistema linealizado por retroalimentación no lineal2/Subsistema físico no lineal /Subsistema térmico ==
  i_qs^r : Inport
  i_ds^r : Inport  Port=2
  i_0s^r : Inport  Port=3
  Tº_amb : Inport  Port=4
  CI = 40ºC : Integrator  InitialCondition=40
  Constant : Constant
  Gain : Gain  Gain=1/C_ts
  Gain1 : Gain  Gain=2
  Gain2 : Gain  Gain=3/2
  Gain3 : Gain  Gain=1/R_ts_amb
  Gain4 : Gain  Gain=alpha_cu
  Gain5 : Gain  Gain=R_s_40
  Product : Product
  Square : Math  Operator=square
  Square1 : Math  Operator=square
  Square2 : Math  Operator=square
  Sum : Sum  Inputs=+++
  Sum1 : Sum  Inputs=|+-
  Sum2 : Sum  Inputs=|+-
  Sum3 : Sum  Inputs=|++
  T_s : Outport
  r_s : Outport  Port=2
  wires:
  CI = 40ºC/1 -> Sum2/2, T_s/1
  Gain/1 -> CI = 40ºC/1
  Sum1/1 -> Gain/1
  i_qs^r/1 -> Square/1
  i_ds^r/1 -> Square1/1
  i_0s^r/1 -> Square2/1
  Square2/1 -> Gain1/1
  Square/1 -> Sum/1
  Square1/1 -> Sum/2
  Gain1/1 -> Sum/3
  Gain5/1 -> r_s/1, Gain2/1
  Gain2/1 -> Product/2
  Sum/1 -> Product/1
  Product/1 -> Sum1/1
  Tº_amb/1 -> Sum2/1
  Sum2/1 -> Gain4/1, Gain3/1
  Gain3/1 -> Sum1/2
  Gain4/1 -> Sum3/1
  Constant/1 -> Sum3/2
  Sum3/1 -> Gain5/1

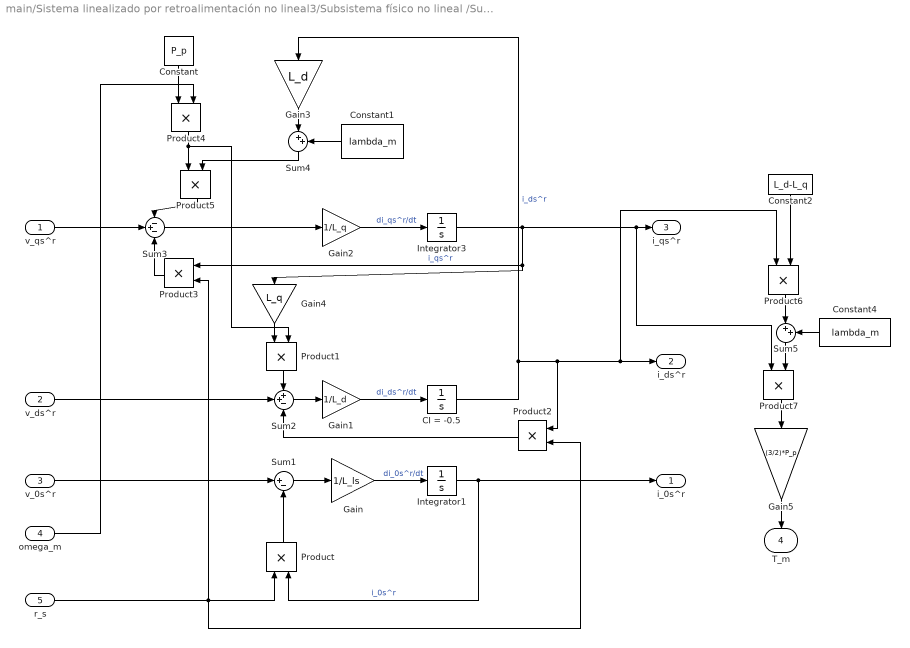
== system main/Sistema linealizado por retroalimentación no lineal3/Subsistema físico no lineal /Subsistema electromagnético ==
  v_qs^r : Inport
  v_ds^r : Inport  Port=2
  v_0s^r : Inport  Port=3
  omega_m : Inport  Port=4
  r_s : Inport  Port=5
  CI = -0.5 : Integrator  InitialCondition=-0.5
  Constant : Constant  Value=P_p
  Constant1 : Constant  Value=lambda_m
  Constant2 : Constant  Value=L_d-L_q
  Constant4 : Constant  Value=lambda_m
  Gain : Gain  Gain=1/L_ls
  Gain1 : Gain  Gain=1/L_d
  Gain2 : Gain  Gain=1/L_q
  Gain3 : Gain  Gain=L_d
  Gain4 : Gain  Gain=L_q
  Gain5 : Gain  Gain=(3/2)*P_p
  Integrator1 : Integrator
  Integrator3 : Integrator
  Product{,1..7} (8 alike) : Product
  Sum1 : Sum  Inputs=|+-
  Sum2 : Sum  Inputs=++-
  Sum3 : Sum  Inputs=-+-
  Sum4 : Sum  Inputs=|++
  Sum5 : Sum  Inputs=|++
  i_0s^r : Outport
  i_ds^r : Outport  Port=2
  i_qs^r : Outport  Port=3
  T_m : Outport  Port=4
  wires:
  Integrator1/1 -> i_0s^r/1, Product/2  "i_0s^r"
  r_s/1 -> Product3/2, Product2/2, Product/1
  Sum1/1 -> Gain/1
  Product/1 -> Sum1/2
  Gain/1 -> Integrator1/1  "di_0s^r/dt"
  v_0s^r/1 -> Sum1/1
  CI = -0.5/1 -> Gain3/1, Product2/1, Product6/1, i_ds^r/1  "i_ds^r"
  Gain1/1 -> CI = -0.5/1  "di_ds^r/dt"
  Sum2/1 -> Gain1/1
  Integrator3/1 -> Product3/1, Gain4/1, Product7/1, i_qs^r/1  "i_qs^r"
  Gain2/1 -> Integrator3/1  "di_qs^r/dt"
  Product3/1 -> Sum3/3
  v_qs^r/1 -> Sum3/2
  Constant/1 -> Product4/1
  omega_m/1 -> Product4/2
  Product4/1 -> Product1/2, Product5/1
  Gain3/1 -> Sum4/1
  Sum4/1 -> Product5/2
  Constant1/1 -> Sum4/2
  Product5/1 -> Sum3/1
  Sum3/1 -> Gain2/1
  v_ds^r/1 -> Sum2/2
  Gain4/1 -> Product1/1
  Product1/1 -> Sum2/1
  Product2/1 -> Sum2/3
  Product6/1 -> Sum5/1
  Constant4/1 -> Sum5/2
  Sum5/1 -> Product7/2
  Product7/1 -> Gain5/1
  Gain5/1 -> T_m/1
  Constant2/1 -> Product6/2

== system main/Sistema linealizado por retroalimentación no lineal3/Subsistema físico no lineal /Subsistema mecánico completo ==
  T_m : Inport
  T_l : Inport  Port=2
  Gain : Gain  Gain=b_m +( b_l / (r^2))
  Gain1 : Gain  Gain=1/r
  Gain2 : Gain  Gain=1/(J_m + J_l / (r^2))
  Sum : Sum  Inputs=-+-
  omega_m(0) = 0 : Integrator
  theta_m(0) = 0 : Integrator
  theta_m(t) : Outport
  omega_m(t) : Outport  Port=2
  wires:
  Gain2/1 -> omega_m(0) = 0/1  "domega_m(t)/dt"
  Gain1/1 -> Sum/1
  theta_m(0) = 0/1 -> theta_m(t)/1  "theta_m(t)"
  omega_m(0) = 0/1 -> omega_m(t)/1, Gain/1, theta_m(0) = 0/1  "omega_m(t)"
  Sum/1 -> Gain2/1
  Gain/1 -> Sum/3
  T_l/1 -> Gain1/1
  T_m/1 -> Sum/2

== system main/Sistema linealizado por retroalimentación no lineal3/Subsistema físico no lineal /Subsistema térmico ==
  i_qs^r : Inport
  i_ds^r : Inport  Port=2
  i_0s^r : Inport  Port=3
  Tº_amb : Inport  Port=4
  CI = 40ºC : Integrator  InitialCondition=40
  Constant : Constant
  Gain : Gain  Gain=1/C_ts
  Gain1 : Gain  Gain=2
  Gain2 : Gain  Gain=3/2
  Gain3 : Gain  Gain=1/R_ts_amb
  Gain4 : Gain  Gain=alpha_cu
  Gain5 : Gain  Gain=R_s_40
  Product : Product
  Square : Math  Operator=square
  Square1 : Math  Operator=square
  Square2 : Math  Operator=square
  Sum : Sum  Inputs=+++
  Sum1 : Sum  Inputs=|+-
  Sum2 : Sum  Inputs=|+-
  Sum3 : Sum  Inputs=|++
  T_s : Outport
  r_s : Outport  Port=2
  wires:
  CI = 40ºC/1 -> Sum2/2, T_s/1
  Gain/1 -> CI = 40ºC/1
  Sum1/1 -> Gain/1
  i_qs^r/1 -> Square/1
  i_ds^r/1 -> Square1/1
  i_0s^r/1 -> Square2/1
  Square2/1 -> Gain1/1
  Square/1 -> Sum/1
  Square1/1 -> Sum/2
  Gain1/1 -> Sum/3
  Gain5/1 -> r_s/1, Gain2/1
  Gain2/1 -> Product/2
  Sum/1 -> Product/1
  Product/1 -> Sum1/1
  Tº_amb/1 -> Sum2/1
  Sum2/1 -> Gain4/1, Gain3/1
  Gain3/1 -> Sum1/2
  Gain4/1 -> Sum3/1
  Constant/1 -> Sum3/2
  Sum3/1 -> Gain5/1

== system main/Sistema linealizado por retroalimentación no lineal4/Subsistema físico no lineal /Subsistema electromagnético ==
  v_qs^r : Inport
  v_ds^r : Inport  Port=2
  v_0s^r : Inport  Port=3
  omega_m : Inport  Port=4
  r_s : Inport  Port=5
  CI = 0 : Integrator
  Constant : Constant  Value=P_p
  Constant1 : Constant  Value=lambda_m
  Constant2 : Constant  Value=L_d-L_q
  Constant4 : Constant  Value=lambda_m
  Gain : Gain  Gain=1/L_ls
  Gain1 : Gain  Gain=1/L_d
  Gain2 : Gain  Gain=1/L_q
  Gain3 : Gain  Gain=L_d
  Gain4 : Gain  Gain=L_q
  Gain5 : Gain  Gain=(3/2)*P_p
  Integrator1 : Integrator
  Integrator3 : Integrator
  Product{,1..7} (8 alike) : Product
  Sum1 : Sum  Inputs=|+-
  Sum2 : Sum  Inputs=++-
  Sum3 : Sum  Inputs=-+-
  Sum4 : Sum  Inputs=|++
  Sum5 : Sum  Inputs=|++
  i_0s^r : Outport
  i_ds^r : Outport  Port=2
  i_qs^r : Outport  Port=3
  T_m : Outport  Port=4
  wires:
  Integrator1/1 -> i_0s^r/1, Product/2  "i_0s^r"
  r_s/1 -> Product3/2, Product2/2, Product/1
  Sum1/1 -> Gain/1
  Product/1 -> Sum1/2
  Gain/1 -> Integrator1/1  "di_0s^r/dt"
  v_0s^r/1 -> Sum1/1
  CI = 0/1 -> Gain3/1, Product2/1, Product6/1, i_ds^r/1  "i_ds^r"
  Gain1/1 -> CI = 0/1  "di_ds^r/dt"
  Sum2/1 -> Gain1/1
  Integrator3/1 -> Product3/1, Gain4/1, Product7/1, i_qs^r/1  "i_qs^r"
  Gain2/1 -> Integrator3/1  "di_qs^r/dt"
  Product3/1 -> Sum3/3
  v_qs^r/1 -> Sum3/2
  Constant/1 -> Product4/1
  omega_m/1 -> Product4/2
  Product4/1 -> Product1/2, Product5/1
  Gain3/1 -> Sum4/1
  Sum4/1 -> Product5/2
  Constant1/1 -> Sum4/2
  Product5/1 -> Sum3/1
  Sum3/1 -> Gain2/1
  v_ds^r/1 -> Sum2/2
  Gain4/1 -> Product1/1
  Product1/1 -> Sum2/1
  Product2/1 -> Sum2/3
  Product6/1 -> Sum5/1
  Constant4/1 -> Sum5/2
  Sum5/1 -> Product7/2
  Product7/1 -> Gain5/1
  Gain5/1 -> T_m/1
  Constant2/1 -> Product6/2

== system main/Sistema linealizado por retroalimentación no lineal4/Subsistema físico no lineal /Subsistema mecánico completo ==
  T_m : Inport
  T_l : Inport  Port=2
  Gain : Gain  Gain=b_m +( b_l / (r^2))
  Gain1 : Gain  Gain=1/r
  Gain2 : Gain  Gain=1/(J_m + J_l / (r^2))
  Sum : Sum  Inputs=-+-
  omega_m(0) = 0 : Integrator
  theta_m(0) = 0 : Integrator
  theta_m(t) : Outport
  omega_m(t) : Outport  Port=2
  wires:
  Gain2/1 -> omega_m(0) = 0/1  "domega_m(t)/dt"
  Gain1/1 -> Sum/1
  theta_m(0) = 0/1 -> theta_m(t)/1  "theta_m(t)"
  omega_m(0) = 0/1 -> omega_m(t)/1, Gain/1, theta_m(0) = 0/1  "omega_m(t)"
  Sum/1 -> Gain2/1
  Gain/1 -> Sum/3
  T_l/1 -> Gain1/1
  T_m/1 -> Sum/2

== system main/Sistema linealizado por retroalimentación no lineal4/Subsistema físico no lineal /Subsistema térmico ==
  i_qs^r : Inport
  i_ds^r : Inport  Port=2
  i_0s^r : Inport  Port=3
  Tº_amb : Inport  Port=4
  CI = 40ºC : Integrator  InitialCondition=40
  Constant : Constant
  Gain : Gain  Gain=1/C_ts
  Gain1 : Gain  Gain=2
  Gain2 : Gain  Gain=3/2
  Gain3 : Gain  Gain=1/R_ts_amb
  Gain4 : Gain  Gain=alpha_cu
  Gain5 : Gain  Gain=R_s_40
  Product : Product
  Square : Math  Operator=square
  Square1 : Math  Operator=square
  Square2 : Math  Operator=square
  Sum : Sum  Inputs=+++
  Sum1 : Sum  Inputs=|+-
  Sum2 : Sum  Inputs=|+-
  Sum3 : Sum  Inputs=|++
  T_s : Outport
  r_s : Outport  Port=2
  wires:
  CI = 40ºC/1 -> Sum2/2, T_s/1
  Gain/1 -> CI = 40ºC/1
  Sum1/1 -> Gain/1
  i_qs^r/1 -> Square/1
  i_ds^r/1 -> Square1/1
  i_0s^r/1 -> Square2/1
  Square2/1 -> Gain1/1
  Square/1 -> Sum/1
  Square1/1 -> Sum/2
  Gain1/1 -> Sum/3
  Gain5/1 -> r_s/1, Gain2/1
  Gain2/1 -> Product/2
  Sum/1 -> Product/1
  Product/1 -> Sum1/1
  Tº_amb/1 -> Sum2/1
  Sum2/1 -> Gain4/1, Gain3/1
  Gain3/1 -> Sum1/2
  Gain4/1 -> Sum3/1
  Constant/1 -> Sum3/2
  Sum3/1 -> Gain5/1

== system main/Sistema linealizado por retroalimentación no lineal5/Subsistema físico no lineal /Subsistema electromagnético ==
  v_qs^r : Inport
  v_ds^r : Inport  Port=2
  v_0s^r : Inport  Port=3
  omega_m : Inport  Port=4
  r_s : Inport  Port=5
  CI = 0 : Integrator
  Constant : Constant  Value=P_p
  Constant1 : Constant  Value=lambda_m
  Constant2 : Constant  Value=L_d-L_q
  Constant4 : Constant  Value=lambda_m
  Gain : Gain  Gain=1/L_ls
  Gain1 : Gain  Gain=1/L_d
  Gain2 : Gain  Gain=1/L_q
  Gain3 : Gain  Gain=L_d
  Gain4 : Gain  Gain=L_q
  Gain5 : Gain  Gain=(3/2)*P_p
  Integrator1 : Integrator
  Integrator3 : Integrator
  Product{,1..7} (8 alike) : Product
  Sum1 : Sum  Inputs=|+-
  Sum2 : Sum  Inputs=++-
  Sum3 : Sum  Inputs=-+-
  Sum4 : Sum  Inputs=|++
  Sum5 : Sum  Inputs=|++
  i_0s^r : Outport
  i_ds^r : Outport  Port=2
  i_qs^r : Outport  Port=3
  T_m : Outport  Port=4
  wires:
  Integrator1/1 -> i_0s^r/1, Product/2  "i_0s^r"
  r_s/1 -> Product3/2, Product2/2, Product/1
  Sum1/1 -> Gain/1
  Product/1 -> Sum1/2
  Gain/1 -> Integrator1/1  "di_0s^r/dt"
  v_0s^r/1 -> Sum1/1
  CI = 0/1 -> Gain3/1, Product2/1, Product6/1, i_ds^r/1  "i_ds^r"
  Gain1/1 -> CI = 0/1  "di_ds^r/dt"
  Sum2/1 -> Gain1/1
  Integrator3/1 -> Product3/1, Gain4/1, Product7/1, i_qs^r/1  "i_qs^r"
  Gain2/1 -> Integrator3/1  "di_qs^r/dt"
  Product3/1 -> Sum3/3
  v_qs^r/1 -> Sum3/2
  Constant/1 -> Product4/1
  omega_m/1 -> Product4/2
  Product4/1 -> Product1/2, Product5/1
  Gain3/1 -> Sum4/1
  Sum4/1 -> Product5/2
  Constant1/1 -> Sum4/2
  Product5/1 -> Sum3/1
  Sum3/1 -> Gain2/1
  v_ds^r/1 -> Sum2/2
  Gain4/1 -> Product1/1
  Product1/1 -> Sum2/1
  Product2/1 -> Sum2/3
  Product6/1 -> Sum5/1
  Constant4/1 -> Sum5/2
  Sum5/1 -> Product7/2
  Product7/1 -> Gain5/1
  Gain5/1 -> T_m/1
  Constant2/1 -> Product6/2

== system main/Sistema linealizado por retroalimentación no lineal5/Subsistema físico no lineal /Subsistema mecánico completo ==
  T_m : Inport
  T_l : Inport  Port=2
  Gain : Gain  Gain=b_m +( b_l / (r^2))
  Gain1 : Gain  Gain=1/r
  Gain2 : Gain  Gain=1/(J_m + J_l / (r^2))
  Sum : Sum  Inputs=-+-
  omega_m(0) = 0 : Integrator
  theta_m(0) = 0 : Integrator
  theta_m(t) : Outport
  omega_m(t) : Outport  Port=2
  wires:
  Gain2/1 -> omega_m(0) = 0/1  "domega_m(t)/dt"
  Gain1/1 -> Sum/1
  theta_m(0) = 0/1 -> theta_m(t)/1  "theta_m(t)"
  omega_m(0) = 0/1 -> omega_m(t)/1, Gain/1, theta_m(0) = 0/1  "omega_m(t)"
  Sum/1 -> Gain2/1
  Gain/1 -> Sum/3
  T_l/1 -> Gain1/1
  T_m/1 -> Sum/2

== system main/Sistema linealizado por retroalimentación no lineal5/Subsistema físico no lineal /Subsistema térmico ==
  i_qs^r : Inport
  i_ds^r : Inport  Port=2
  i_0s^r : Inport  Port=3
  Tº_amb : Inport  Port=4
  CI = 40ºC : Integrator  InitialCondition=40
  Constant : Constant
  Gain : Gain  Gain=1/C_ts
  Gain1 : Gain  Gain=2
  Gain2 : Gain  Gain=3/2
  Gain3 : Gain  Gain=1/R_ts_amb
  Gain4 : Gain  Gain=alpha_cu
  Gain5 : Gain  Gain=R_s_40
  Product : Product
  Square : Math  Operator=square
  Square1 : Math  Operator=square
  Square2 : Math  Operator=square
  Sum : Sum  Inputs=+++
  Sum1 : Sum  Inputs=|+-
  Sum2 : Sum  Inputs=|+-
  Sum3 : Sum  Inputs=|++
  T_s : Outport
  r_s : Outport  Port=2
  wires:
  CI = 40ºC/1 -> Sum2/2, T_s/1
  Gain/1 -> CI = 40ºC/1
  Sum1/1 -> Gain/1
  i_qs^r/1 -> Square/1
  i_ds^r/1 -> Square1/1
  i_0s^r/1 -> Square2/1
  Square2/1 -> Gain1/1
  Square/1 -> Sum/1
  Square1/1 -> Sum/2
  Gain1/1 -> Sum/3
  Gain5/1 -> r_s/1, Gain2/1
  Gain2/1 -> Product/2
  Sum/1 -> Product/1
  Product/1 -> Sum1/1
  Tº_amb/1 -> Sum2/1
  Sum2/1 -> Gain4/1, Gain3/1
  Gain3/1 -> Sum1/2
  Gain4/1 -> Sum3/1
  Constant/1 -> Sum3/2
  Sum3/1 -> Gain5/1

== matlab function main/Sistema lineal equivalente1/TI_PARK1 ==
  data: fqs input; fas output; fds input; f0s input; theta_r input; fbs output; fcs output
function [fas, fbs, fcs] = TI_PARK(fqs, fds, f0s , theta_r)

    fqd0s = [fqs; fds; f0s];

    Ks = [cos(theta_r)         sin(theta_r)             1
          cos(theta_r - 2*pi/3) sin(theta_r - 2*pi/3)    1
          cos(theta_r + 2*pi/3) sin(theta_r + 2*pi/3)    1];

    fabcs = Ks * fqd0s;

    fas = fabcs(1);
    fbs = fabcs(2);
    fcs = fabcs(3);

end

== matlab function main/Sistema completo/TI_PARK ==
  data: fqs input; fas output; fds input; f0s input; theta_r input; fbs output; fcs output
function [fas, fbs, fcs] = TI_PARK(fqs, fds, f0s , theta_r)

    fqd0s = [fqs; fds; f0s];

    Ks = [cos(theta_r)         sin(theta_r)             1
          cos(theta_r - 2*pi/3) sin(theta_r - 2*pi/3)    1
          cos(theta_r + 2*pi/3) sin(theta_r + 2*pi/3)    1];

    fabcs = Ks * fqd0s;

    fas = fabcs(1);
    fbs = fabcs(2);
    fcs = fabcs(3);

end
